simulink model "Lab2_PID"  (R2021a)
settings: Solver=VariableStepAuto  StartTime=0.0  StopTime=10.0  FixedStep=1e-3  MaxStep=1e-3  RelTol=1e-3
settings Model: Creator=maria  LastModifiedBy=maria

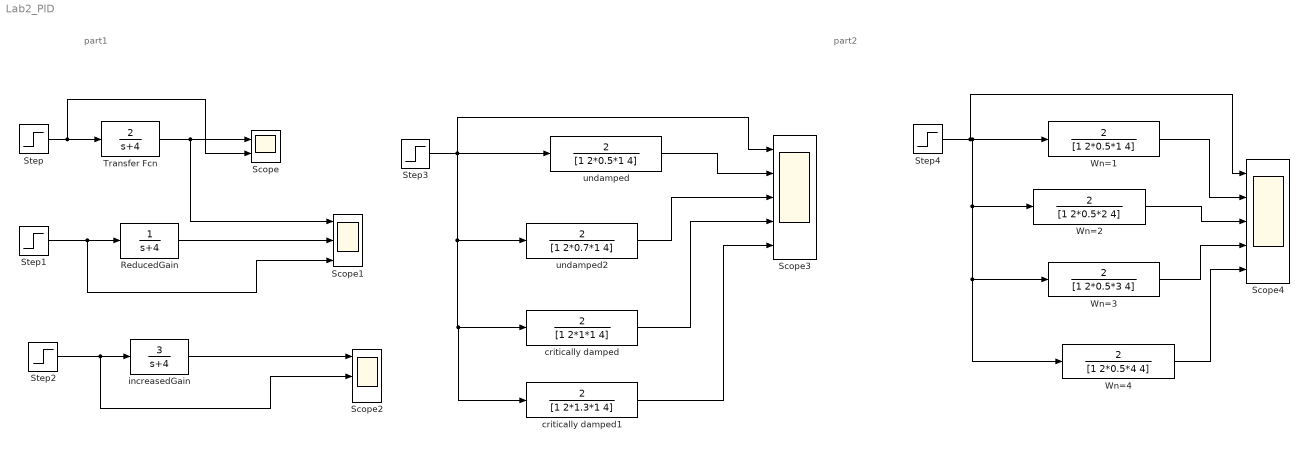
== system Lab2_PID ==
  note: part1
  note: part2
  ReducedGain : TransferFcn  Denominator=[1 4]
  Scope : Scope  NumInputPorts=2
  Scope1 : Scope  NumInputPorts=3
  Scope2 : Scope  NumInputPorts=3
  Scope3 : Scope  NumInputPorts=5
  Scope4 : Scope  NumInputPorts=5
  Step : Step  SampleTime=0
  Step1 : Step  SampleTime=0
  Step2 : Step  Time=5  After=0.5  SampleTime=0
  Step3 : Step  After=0.5  SampleTime=0
  Step4 : Step  After=0.5  SampleTime=0
  Transfer Fcn : TransferFcn  Numerator=[2]  Denominator=[1 4]
  Wn=1 : TransferFcn  Numerator=[2]  Denominator=[1 2*0.5*1 4]
  Wn=2 : TransferFcn  Numerator=[2]  Denominator=[1 2*0.5*2 4]
  Wn=3 : TransferFcn  Numerator=[2]  Denominator=[1 2*0.5*3 4]
  Wn=4 : TransferFcn  Numerator=[2]  Denominator=[1 2*0.5*4 4]
  critically damped : TransferFcn  Numerator=[2]  Denominator=[1 2*1*1 4]
  critically damped1 : TransferFcn  Numerator=[2]  Denominator=[1 2*1.3*1 4]
  increasedGain : TransferFcn  Numerator=[3]  Denominator=[1 4]
  undamped : TransferFcn  Numerator=[2]  Denominator=[1 2*0.5*1 4]
  undamped2 : TransferFcn  Numerator=[2]  Denominator=[1 2*0.7*1 4]
  wires:
  Transfer Fcn/1 -> Scope1/1, Scope/1
  Step/1 -> Scope/2, Transfer Fcn/1
  Step1/1 -> Scope1/3, ReducedGain/1
  ReducedGain/1 -> Scope1/2
  Step2/1 -> Scope2/2, increasedGain/1
  increasedGain/1 -> Scope2/1
  Step3/1 -> critically damped1/1, critically damped/1, undamped2/1, Scope3/1, undamped/1
  undamped2/1 -> Scope3/3
  undamped/1 -> Scope3/2
  critically damped/1 -> Scope3/4
  critically damped1/1 -> Scope3/5
  Wn=1/1 -> Scope4/2
  Wn=2/1 -> Scope4/3
  Wn=3/1 -> Scope4/4
  Wn=4/1 -> Scope4/5
  Step4/1 -> Scope4/1, Wn=1/1, Wn=4/1, Wn=3/1, Wn=2/1
